simulink model "BehPlantIronLadle"  (R2026a)
settings: Solver=VariableStepAuto  StopTime=14400
undefined symbols (not defined in the file): IL_Resupply_bph, IL_StaticPower_kW
settings Model: DataDictionary=BehParamsIronLadle.sldd  Creator=sarah  LastModifiedBy=sarah

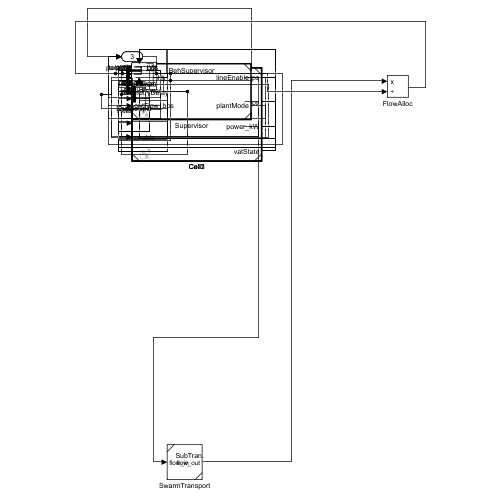
[thumbnail: Simulink's stored preview of the top-level diagram]
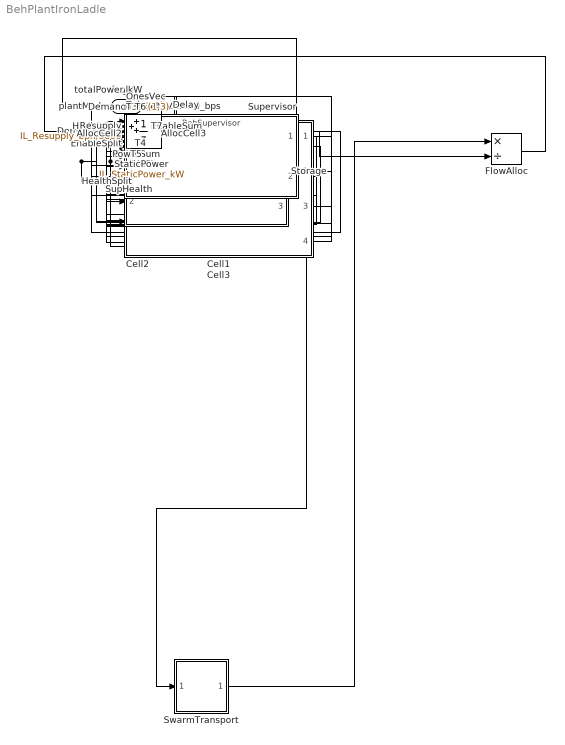
== system BehPlantIronLadle ==
  faults : Inport  PortDimensions=3
  AllocCell1 : Product
  AllocCell2 : Product
  AllocCell3 : Product
  Cell1 : ModelReference  ModelNameDialog=BehProductionCell  UsingDefaultArgumentValue=0,0,0,0,0,0,0,0,0,0,0,0,0  SimulationMode=Normal  ModelReferenceVersion=1.4
  Cell2 : ModelReference  ModelNameDialog=BehProductionCell  UsingDefaultArgumentValue=0,0,0,0,0,0,0,0,0,0,0,0,0  SimulationMode=Normal  ModelReferenceVersion=1.4
  Cell3 : ModelReference  ModelNameDialog=BehProductionCell  UsingDefaultArgumentValue=0,0,0,0,0,0,0,0,0,0,0,0,0  SimulationMode=Normal  ModelReferenceVersion=1.4
  CellMerge : Sum  Inputs=+++
  CellPower : Sum  Inputs=+++
  DemandDelay : UnitDelay
  DemandSum : Sum  Inputs=+++
  EnableFloor : Saturate  UpperLimit=inf  LowerLimit=1
  EnableSplit : Demux
  EnableSum : Sum  Inputs=+++
  FlowAlloc : Product  Inputs=*/
  HealthCalc : Sum  Inputs=+-
  HealthSplit : Demux  Outputs=3
  One : Constant
  OnesVec : Constant  Value=ones(1,3)
  PowerSum : Sum  Inputs=|++
  Resupply : Constant  Value=IL_Resupply_bph/3600
  StaticPower : Constant  Value=IL_StaticPower_kW
  Storage : ModelReference  ModelNameDialog=BehStorage  UsingDefaultArgumentValue=0,0  SimulationMode=Normal  ModelReferenceVersion=1.2
  SupHealth : Mux
  Supervisor : ModelReference  ModelNameDialog=BehSupervisor  ParameterArgumentNames=NumLines  ParameterArgumentValues=IL_NumLines  UsingDefaultArgumentValue=0  SimulationMode=Normal  ModelReferenceVersion=1.3
  SwarmTransport : Subsystem  ReferencedSubsystem=SubTransport
  T{1..7} (7 alike) : Terminator
  TelemetryDelay : UnitDelay
  packedFlow_bps : Outport
  plantMode : Outport  Port=2
  totalPower_kW : Outport  Port=3
  wires:
  OnesVec/1 -> HealthCalc/1
  faults/1 -> HealthCalc/2
  HealthCalc/1 -> HealthSplit/1
  Resupply/1 -> Storage/1
  Cell1/2 -> DemandSum/1
  Cell2/2 -> DemandSum/2
  Cell3/2 -> DemandSum/3
  DemandSum/1 -> DemandDelay/1
  DemandDelay/1 -> Storage/2
  Storage/1 -> SwarmTransport/1
  EnableSplit/1 -> Cell1/2, AllocCell1/2, EnableSum/1
  EnableSplit/2 -> Cell2/2, EnableSum/2, AllocCell2/2
  EnableSplit/3 -> Cell3/2, AllocCell3/2, EnableSum/3
  EnableSum/1 -> EnableFloor/1
  SwarmTransport/1 -> FlowAlloc/1
  EnableFloor/1 -> FlowAlloc/2
  FlowAlloc/1 -> AllocCell3/1, AllocCell2/1, AllocCell1/1
  AllocCell1/1 -> Cell1/1
  AllocCell2/1 -> Cell2/1
  AllocCell3/1 -> Cell3/1
  Cell1/1 -> CellMerge/1
  Cell2/1 -> CellMerge/2
  Cell3/1 -> CellMerge/3
  CellMerge/1 -> TelemetryDelay/1, packedFlow_bps/1
  HealthSplit/1 -> SupHealth/1
  HealthSplit/2 -> SupHealth/2
  HealthSplit/3 -> SupHealth/3
  One/1 -> T7/1, SupHealth/4
  SupHealth/1 -> Supervisor/1
  TelemetryDelay/1 -> Supervisor/2
  Supervisor/1 -> EnableSplit/1
  Supervisor/2 -> plantMode/1
  Cell1/3 -> CellPower/1
  Cell2/3 -> CellPower/2
  Cell3/3 -> CellPower/3
  CellPower/1 -> PowerSum/1
  StaticPower/1 -> PowerSum/2
  PowerSum/1 -> totalPower_kW/1
  Storage/2 -> T1/1
  Storage/3 -> T2/1
  Cell1/4 -> T3/1
  Cell2/4 -> T4/1
  Cell3/4 -> T5/1
  EnableSplit/4 -> T6/1
